simulink model "RoboticArm"  (R2023b)
settings: Solver=ode23t  StartTime=0.0  StopTime=100  RelTol=1e-3
model workspace: external: MATLAB File D:\Projects\RoboticArm\RoboticArm_DataFile1.m (data not in the file)
undefined symbols (not defined in the file or in its folder): dfdbk, dFilt, nfdbk, nFilt, smiData, ST, X, Y, Z
libraries: sm_lib x180, fl_lib x129, nesl_utility x69, ee_lib x39, slpidlib x25, simulink x18, SignalEditorBlockLib x1
(part 2 of 7)

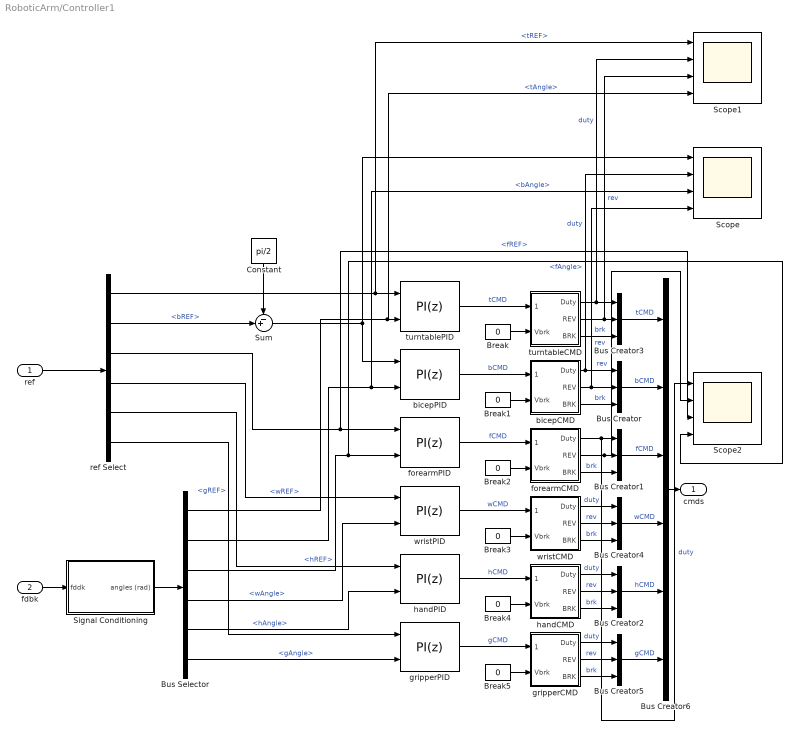
== system RoboticArm/Controller1 ==
  ref : Inport
  fdbk : Inport  Port=2
  Break{,1..5} (6 alike) : Constant  Value=0
  Bus Creator{,1..5} (6 alike) : BusCreator  Inputs=3
  Bus Creator6 : BusCreator  Inputs=6
  Bus Selector : BusSelector  OutputSignals=tAngle,bAngle,fAngle,wAngle,hAngle,gAngle
  Constant : Constant  Value=pi/2
  Scope : Scope  NumInputPorts=4
  Scope1 : Scope  NumInputPorts=4
  Scope2 : Scope  NumInputPorts=4
  Signal Conditioning : Subsystem
  Sum : Sum  Inputs=-+|
  bicepCMD : Subsystem
  bicepPID : slpidlib/PID Controller (2DOF)  Controller=PI  Form=Parallel  TimeDomain=Discrete-time  UseExternalTs=off  SampleTime=ST  IntegratorMethod=Forward Euler  FilterMethod=Backward Euler  ControllerParametersSource=internal  P=6  I=3  UseKiTs=off  D=2.0  N=25  UseFilter=on  b=1  c=1  TunerSelectOption=Transfer Function Based (PID Tuner App)  InitialConditionSource=internal  InitialConditionForIntegrator=0  InitialConditionForFilter=0  DifferentiatorICPrevScaledInput=0  ExternalReset=none  TrackingMode=off  Kt=1  LimitOutput=on  SatLimitsSource=internal  UpperSaturationLimit=5  LowerSaturationLimit=-5  LinearizeAsGain=on  AntiWindupMode=clamping  Kb=1  LimitIntegrator=off  UpperIntegratorSaturationLimit=inf  LowerIntegratorSaturationLimit=-inf  POutMin=[]  POutMax=[]  IOutMin=[]  IOutMax=[]  DOutMin=[]  DOutMax=[]  NOutMin=[]  NOutMax=[]  bOutMin=[]  bOutMax=[]  cOutMin=[]  cOutMax=[]  SumOutMin=[]  SumOutMax=[]  SaturationOutMin=[]  SaturationOutMax=[]  PParamMin=[]  PParamMax=[]  IParamMin=[]  IParamMax=[]  DParamMin=[]  DParamMax=[]  NParamMin=[]  NParamMax=[]  bParamMin=[]  bParamMax=[]  cParamMin=[]  cParamMax=[]  KbParamMin=[]  KbParamMax=[]  KtParamMin=[]  KtParamMax=[]  KbOutMin=[]  KbOutMax=[]  KtOutMin=[]  KtOutMax=[]  IntegratorOutMin=[]  IntegratorOutMax=[]  FilterOutMin=[]  FilterOutMax=[]  SumI1OutMin=[]  SumI1OutMax=[]  SumI2OutMin=[]  SumI2OutMax=[]  SumI3OutMin=[]  SumI3OutMax=[]  SumI4OutMin=[]  SumI4OutMax=[]  SumDOutMin=[]  SumDOutMax=[]  Sum1OutMin=[]  Sum1OutMax=[]  Sum2OutMin=[]  Sum2OutMax=[]  Sum3OutMin=[]  Sum3OutMax=[]  DifferentiatorOutMin=[]  DifferentiatorOutMax=[]  FilterDiffOutCoefMin=[]  FilterDiffOutCoefMax=[]  ReciprocalOutMin=[]  ReciprocalOutMax=[]  SumDenOutMin=[]  SumDenOutMax=[]  SumNumOutMin=[]  SumNumOutMax=[]  DivideOutMin=[]  DivideOutMax=[]  UdiffTsProdOutMin=[]  UdiffTsProdOutMax=[]  NTsProdOutMin=[]  NTsProdOutMax=[]  UintegralTsProdOutMin=[]  UintegralTsProdOutMax=[]  UngainTsProdOutMin=[]  UngainTsProdOutMax=[]  ClampingZeroOutDataTypeStr=Inherit: Inherit via back propagation  ClampingZeroOutMin=[]  ClampingZeroOutMax=[]  FilterDenConstantOutDataTypeStr=Inherit: Inherit via back propagation  FilterDenConstantOutMin=[]  FilterDenConstantOutMax=[]  PCopyOutDataTypeStr=Inherit: Inherit via back propagation  PCopyOutMin=[]  PCopyOutMax=[]  NCopyOutDataTypeStr=Inherit: Inherit via back propagation  NCopyOutMin=[]  NCopyOutMax=[]  IntegratorContinuousStateAttributes=''  IntegratorStateMustResolveToSignalObject=off  IntegratorRTWStateStorageClass=Auto  FilterContinuousStateAttributes=''  FilterStateMustResolveToSignalObject=off  FilterRTWStateStorageClass=Auto  ParallelPVariant=InternalParameters  IdealPVariant=Disabled  IVariant=InternalParameters  DVariant=Disabled  bVariant=InternalParameters  cVariant=Disabled  IntegratorVariant=Discrete  SatVariant=Enabled  AWVariant=DiscClampingParallel  PCopyVariant=Disabled  TRVariant=Disabled  FdbkBlocksVariant=Forward  IdealPFdbkVariant=Disabled  SatFdbkVariant=Disabled  DerivativeFilterVariant=Disabled  NVariant=Disabled  NCopyVariant=Disabled_SignalSpec  FilterICVariant=Disabled  IntegratorICVariant=InternalICs  ExternalResetVariant=Disabled  TRSumVariant=Passthrough  SumFdbkVariant=Disabled  SumVariant=Sum_PI  TsampFilterVariant=InternalTs  TsampNgainVariant=Passthrough  TsampIntegralVariant=Disabled_SignalSpec  ExternalSaturationOutDataTypeStr=Inherit: Same as second input
  forearmCMD : Subsystem
  forearmPID : slpidlib/PID Controller (2DOF)  Controller=PI  Form=Parallel  TimeDomain=Discrete-time  UseExternalTs=off  SampleTime=ST  IntegratorMethod=Forward Euler  FilterMethod=Backward Euler  ControllerParametersSource=internal  P=6  I=3  UseKiTs=off  D=2.0  N=25  UseFilter=on  b=1  c=1  TunerSelectOption=Transfer Function Based (PID Tuner App)  InitialConditionSource=internal  InitialConditionForIntegrator=0  InitialConditionForFilter=0  DifferentiatorICPrevScaledInput=0  ExternalReset=none  TrackingMode=off  Kt=1  LimitOutput=on  SatLimitsSource=internal  UpperSaturationLimit=5  LowerSaturationLimit=-5  LinearizeAsGain=on  AntiWindupMode=clamping  Kb=1  LimitIntegrator=off  UpperIntegratorSaturationLimit=inf  LowerIntegratorSaturationLimit=-inf  POutMin=[]  POutMax=[]  IOutMin=[]  IOutMax=[]  DOutMin=[]  DOutMax=[]  NOutMin=[]  NOutMax=[]  bOutMin=[]  bOutMax=[]  cOutMin=[]  cOutMax=[]  SumOutMin=[]  SumOutMax=[]  SaturationOutMin=[]  SaturationOutMax=[]  PParamMin=[]  PParamMax=[]  IParamMin=[]  IParamMax=[]  DParamMin=[]  DParamMax=[]  NParamMin=[]  NParamMax=[]  bParamMin=[]  bParamMax=[]  cParamMin=[]  cParamMax=[]  KbParamMin=[]  KbParamMax=[]  KtParamMin=[]  KtParamMax=[]  KbOutMin=[]  KbOutMax=[]  KtOutMin=[]  KtOutMax=[]  IntegratorOutMin=[]  IntegratorOutMax=[]  FilterOutMin=[]  FilterOutMax=[]  SumI1OutMin=[]  SumI1OutMax=[]  SumI2OutMin=[]  SumI2OutMax=[]  SumI3OutMin=[]  SumI3OutMax=[]  SumI4OutMin=[]  SumI4OutMax=[]  SumDOutMin=[]  SumDOutMax=[]  Sum1OutMin=[]  Sum1OutMax=[]  Sum2OutMin=[]  Sum2OutMax=[]  Sum3OutMin=[]  Sum3OutMax=[]  DifferentiatorOutMin=[]  DifferentiatorOutMax=[]  FilterDiffOutCoefMin=[]  FilterDiffOutCoefMax=[]  ReciprocalOutMin=[]  ReciprocalOutMax=[]  SumDenOutMin=[]  SumDenOutMax=[]  SumNumOutMin=[]  SumNumOutMax=[]  DivideOutMin=[]  DivideOutMax=[]  UdiffTsProdOutMin=[]  UdiffTsProdOutMax=[]  NTsProdOutMin=[]  NTsProdOutMax=[]  UintegralTsProdOutMin=[]  UintegralTsProdOutMax=[]  UngainTsProdOutMin=[]  UngainTsProdOutMax=[]  ClampingZeroOutDataTypeStr=Inherit: Inherit via back propagation  ClampingZeroOutMin=[]  ClampingZeroOutMax=[]  FilterDenConstantOutDataTypeStr=Inherit: Inherit via back propagation  FilterDenConstantOutMin=[]  FilterDenConstantOutMax=[]  PCopyOutDataTypeStr=Inherit: Inherit via back propagation  PCopyOutMin=[]  PCopyOutMax=[]  NCopyOutDataTypeStr=Inherit: Inherit via back propagation  NCopyOutMin=[]  NCopyOutMax=[]  IntegratorContinuousStateAttributes=''  IntegratorStateMustResolveToSignalObject=off  IntegratorRTWStateStorageClass=Auto  FilterContinuousStateAttributes=''  FilterStateMustResolveToSignalObject=off  FilterRTWStateStorageClass=Auto  ParallelPVariant=InternalParameters  IdealPVariant=Disabled  IVariant=InternalParameters  DVariant=Disabled  bVariant=InternalParameters  cVariant=Disabled  IntegratorVariant=Discrete  SatVariant=Enabled  AWVariant=DiscClampingParallel  PCopyVariant=Disabled  TRVariant=Disabled  FdbkBlocksVariant=Forward  IdealPFdbkVariant=Disabled  SatFdbkVariant=Disabled  DerivativeFilterVariant=Disabled  NVariant=Disabled  NCopyVariant=Disabled_SignalSpec  FilterICVariant=Disabled  IntegratorICVariant=InternalICs  ExternalResetVariant=Disabled  TRSumVariant=Passthrough  SumFdbkVariant=Disabled  SumVariant=Sum_PI  TsampFilterVariant=InternalTs  TsampNgainVariant=Passthrough  TsampIntegralVariant=Disabled_SignalSpec  ExternalSaturationOutDataTypeStr=Inherit: Same as second input
  gripperCMD : Subsystem
  gripperPID : slpidlib/PID Controller (2DOF)  Controller=PI  Form=Parallel  TimeDomain=Discrete-time  UseExternalTs=off  SampleTime=ST  IntegratorMethod=Forward Euler  FilterMethod=Backward Euler  ControllerParametersSource=internal  P=3  I=3  UseKiTs=off  D=2.0  N=25  UseFilter=on  b=1  c=1  TunerSelectOption=Transfer Function Based (PID Tuner App)  InitialConditionSource=internal  InitialConditionForIntegrator=0  InitialConditionForFilter=0  DifferentiatorICPrevScaledInput=0  ExternalReset=none  TrackingMode=off  Kt=1  LimitOutput=on  SatLimitsSource=internal  UpperSaturationLimit=5  LowerSaturationLimit=-5  LinearizeAsGain=on  AntiWindupMode=clamping  Kb=1  LimitIntegrator=off  UpperIntegratorSaturationLimit=inf  LowerIntegratorSaturationLimit=-inf  POutMin=[]  POutMax=[]  IOutMin=[]  IOutMax=[]  DOutMin=[]  DOutMax=[]  NOutMin=[]  NOutMax=[]  bOutMin=[]  bOutMax=[]  cOutMin=[]  cOutMax=[]  SumOutMin=[]  SumOutMax=[]  SaturationOutMin=[]  SaturationOutMax=[]  PParamMin=[]  PParamMax=[]  IParamMin=[]  IParamMax=[]  DParamMin=[]  DParamMax=[]  NParamMin=[]  NParamMax=[]  bParamMin=[]  bParamMax=[]  cParamMin=[]  cParamMax=[]  KbParamMin=[]  KbParamMax=[]  KtParamMin=[]  KtParamMax=[]  KbOutMin=[]  KbOutMax=[]  KtOutMin=[]  KtOutMax=[]  IntegratorOutMin=[]  IntegratorOutMax=[]  FilterOutMin=[]  FilterOutMax=[]  SumI1OutMin=[]  SumI1OutMax=[]  SumI2OutMin=[]  SumI2OutMax=[]  SumI3OutMin=[]  SumI3OutMax=[]  SumI4OutMin=[]  SumI4OutMax=[]  SumDOutMin=[]  SumDOutMax=[]  Sum1OutMin=[]  Sum1OutMax=[]  Sum2OutMin=[]  Sum2OutMax=[]  Sum3OutMin=[]  Sum3OutMax=[]  DifferentiatorOutMin=[]  DifferentiatorOutMax=[]  FilterDiffOutCoefMin=[]  FilterDiffOutCoefMax=[]  ReciprocalOutMin=[]  ReciprocalOutMax=[]  SumDenOutMin=[]  SumDenOutMax=[]  SumNumOutMin=[]  SumNumOutMax=[]  DivideOutMin=[]  DivideOutMax=[]  UdiffTsProdOutMin=[]  UdiffTsProdOutMax=[]  NTsProdOutMin=[]  NTsProdOutMax=[]  UintegralTsProdOutMin=[]  UintegralTsProdOutMax=[]  UngainTsProdOutMin=[]  UngainTsProdOutMax=[]  ClampingZeroOutDataTypeStr=Inherit: Inherit via back propagation  ClampingZeroOutMin=[]  ClampingZeroOutMax=[]  FilterDenConstantOutDataTypeStr=Inherit: Inherit via back propagation  FilterDenConstantOutMin=[]  FilterDenConstantOutMax=[]  PCopyOutDataTypeStr=Inherit: Inherit via back propagation  PCopyOutMin=[]  PCopyOutMax=[]  NCopyOutDataTypeStr=Inherit: Inherit via back propagation  NCopyOutMin=[]  NCopyOutMax=[]  IntegratorContinuousStateAttributes=''  IntegratorStateMustResolveToSignalObject=off  IntegratorRTWStateStorageClass=Auto  FilterContinuousStateAttributes=''  FilterStateMustResolveToSignalObject=off  FilterRTWStateStorageClass=Auto  ParallelPVariant=InternalParameters  IdealPVariant=Disabled  IVariant=InternalParameters  DVariant=Disabled  bVariant=InternalParameters  cVariant=Disabled  IntegratorVariant=Discrete  SatVariant=Enabled  AWVariant=DiscClampingParallel  PCopyVariant=Disabled  TRVariant=Disabled  FdbkBlocksVariant=Forward  IdealPFdbkVariant=Disabled  SatFdbkVariant=Disabled  DerivativeFilterVariant=Disabled  NVariant=Disabled  NCopyVariant=Disabled_SignalSpec  FilterICVariant=Disabled  IntegratorICVariant=InternalICs  ExternalResetVariant=Disabled  TRSumVariant=Passthrough  SumFdbkVariant=Disabled  SumVariant=Sum_PI  TsampFilterVariant=InternalTs  TsampNgainVariant=Passthrough  TsampIntegralVariant=Disabled_SignalSpec  ExternalSaturationOutDataTypeStr=Inherit: Same as second input
  handCMD : Subsystem
  handPID : slpidlib/PID Controller (2DOF)  Controller=PI  Form=Parallel  TimeDomain=Discrete-time  UseExternalTs=off  SampleTime=ST  IntegratorMethod=Forward Euler  FilterMethod=Backward Euler  ControllerParametersSource=internal  P=3  I=3  UseKiTs=off  D=2.0  N=25  UseFilter=on  b=1  c=1  TunerSelectOption=Transfer Function Based (PID Tuner App)  InitialConditionSource=internal  InitialConditionForIntegrator=0  InitialConditionForFilter=0  DifferentiatorICPrevScaledInput=0  ExternalReset=none  TrackingMode=off  Kt=1  LimitOutput=on  SatLimitsSource=internal  UpperSaturationLimit=5  LowerSaturationLimit=-5  LinearizeAsGain=on  AntiWindupMode=clamping  Kb=1  LimitIntegrator=off  UpperIntegratorSaturationLimit=inf  LowerIntegratorSaturationLimit=-inf  POutMin=[]  POutMax=[]  IOutMin=[]  IOutMax=[]  DOutMin=[]  DOutMax=[]  NOutMin=[]  NOutMax=[]  bOutMin=[]  bOutMax=[]  cOutMin=[]  cOutMax=[]  SumOutMin=[]  SumOutMax=[]  SaturationOutMin=[]  SaturationOutMax=[]  PParamMin=[]  PParamMax=[]  IParamMin=[]  IParamMax=[]  DParamMin=[]  DParamMax=[]  NParamMin=[]  NParamMax=[]  bParamMin=[]  bParamMax=[]  cParamMin=[]  cParamMax=[]  KbParamMin=[]  KbParamMax=[]  KtParamMin=[]  KtParamMax=[]  KbOutMin=[]  KbOutMax=[]  KtOutMin=[]  KtOutMax=[]  IntegratorOutMin=[]  IntegratorOutMax=[]  FilterOutMin=[]  FilterOutMax=[]  SumI1OutMin=[]  SumI1OutMax=[]  SumI2OutMin=[]  SumI2OutMax=[]  SumI3OutMin=[]  SumI3OutMax=[]  SumI4OutMin=[]  SumI4OutMax=[]  SumDOutMin=[]  SumDOutMax=[]  Sum1OutMin=[]  Sum1OutMax=[]  Sum2OutMin=[]  Sum2OutMax=[]  Sum3OutMin=[]  Sum3OutMax=[]  DifferentiatorOutMin=[]  DifferentiatorOutMax=[]  FilterDiffOutCoefMin=[]  FilterDiffOutCoefMax=[]  ReciprocalOutMin=[]  ReciprocalOutMax=[]  SumDenOutMin=[]  SumDenOutMax=[]  SumNumOutMin=[]  SumNumOutMax=[]  DivideOutMin=[]  DivideOutMax=[]  UdiffTsProdOutMin=[]  UdiffTsProdOutMax=[]  NTsProdOutMin=[]  NTsProdOutMax=[]  UintegralTsProdOutMin=[]  UintegralTsProdOutMax=[]  UngainTsProdOutMin=[]  UngainTsProdOutMax=[]  ClampingZeroOutDataTypeStr=Inherit: Inherit via back propagation  ClampingZeroOutMin=[]  ClampingZeroOutMax=[]  FilterDenConstantOutDataTypeStr=Inherit: Inherit via back propagation  FilterDenConstantOutMin=[]  FilterDenConstantOutMax=[]  PCopyOutDataTypeStr=Inherit: Inherit via back propagation  PCopyOutMin=[]  PCopyOutMax=[]  NCopyOutDataTypeStr=Inherit: Inherit via back propagation  NCopyOutMin=[]  NCopyOutMax=[]  IntegratorContinuousStateAttributes=''  IntegratorStateMustResolveToSignalObject=off  IntegratorRTWStateStorageClass=Auto  FilterContinuousStateAttributes=''  FilterStateMustResolveToSignalObject=off  FilterRTWStateStorageClass=Auto  ParallelPVariant=InternalParameters  IdealPVariant=Disabled  IVariant=InternalParameters  DVariant=Disabled  bVariant=InternalParameters  cVariant=Disabled  IntegratorVariant=Discrete  SatVariant=Enabled  AWVariant=DiscClampingParallel  PCopyVariant=Disabled  TRVariant=Disabled  FdbkBlocksVariant=Forward  IdealPFdbkVariant=Disabled  SatFdbkVariant=Disabled  DerivativeFilterVariant=Disabled  NVariant=Disabled  NCopyVariant=Disabled_SignalSpec  FilterICVariant=Disabled  IntegratorICVariant=InternalICs  ExternalResetVariant=Disabled  TRSumVariant=Passthrough  SumFdbkVariant=Disabled  SumVariant=Sum_PI  TsampFilterVariant=InternalTs  TsampNgainVariant=Passthrough  TsampIntegralVariant=Disabled_SignalSpec  ExternalSaturationOutDataTypeStr=Inherit: Same as second input
  ref Select : BusSelector  OutputSignals=tREF,bREF,fREF,wREF,hREF,gREF
  turntableCMD : Subsystem
  turntablePID : slpidlib/PID Controller (2DOF)  Controller=PI  Form=Parallel  TimeDomain=Discrete-time  UseExternalTs=off  SampleTime=ST  IntegratorMethod=Forward Euler  FilterMethod=Backward Euler  ControllerParametersSource=internal  P=3  I=3  UseKiTs=off  D=2.0  N=25  UseFilter=on  b=1  c=1  TunerSelectOption=Transfer Function Based (PID Tuner App)  InitialConditionSource=internal  InitialConditionForIntegrator=0  InitialConditionForFilter=0  DifferentiatorICPrevScaledInput=0  ExternalReset=none  TrackingMode=off  Kt=1  LimitOutput=on  SatLimitsSource=internal  UpperSaturationLimit=5  LowerSaturationLimit=-5  LinearizeAsGain=on  AntiWindupMode=clamping  Kb=1  LimitIntegrator=off  UpperIntegratorSaturationLimit=inf  LowerIntegratorSaturationLimit=-inf  POutMin=[]  POutMax=[]  IOutMin=[]  IOutMax=[]  DOutMin=[]  DOutMax=[]  NOutMin=[]  NOutMax=[]  bOutMin=[]  bOutMax=[]  cOutMin=[]  cOutMax=[]  SumOutMin=[]  SumOutMax=[]  SaturationOutMin=[]  SaturationOutMax=[]  PParamMin=[]  PParamMax=[]  IParamMin=[]  IParamMax=[]  DParamMin=[]  DParamMax=[]  NParamMin=[]  NParamMax=[]  bParamMin=[]  bParamMax=[]  cParamMin=[]  cParamMax=[]  KbParamMin=[]  KbParamMax=[]  KtParamMin=[]  KtParamMax=[]  KbOutMin=[]  KbOutMax=[]  KtOutMin=[]  KtOutMax=[]  IntegratorOutMin=[]  IntegratorOutMax=[]  FilterOutMin=[]  FilterOutMax=[]  SumI1OutMin=[]  SumI1OutMax=[]  SumI2OutMin=[]  SumI2OutMax=[]  SumI3OutMin=[]  SumI3OutMax=[]  SumI4OutMin=[]  SumI4OutMax=[]  SumDOutMin=[]  SumDOutMax=[]  Sum1OutMin=[]  Sum1OutMax=[]  Sum2OutMin=[]  Sum2OutMax=[]  Sum3OutMin=[]  Sum3OutMax=[]  DifferentiatorOutMin=[]  DifferentiatorOutMax=[]  FilterDiffOutCoefMin=[]  FilterDiffOutCoefMax=[]  ReciprocalOutMin=[]  ReciprocalOutMax=[]  SumDenOutMin=[]  SumDenOutMax=[]  SumNumOutMin=[]  SumNumOutMax=[]  DivideOutMin=[]  DivideOutMax=[]  UdiffTsProdOutMin=[]  UdiffTsProdOutMax=[]  NTsProdOutMin=[]  NTsProdOutMax=[]  UintegralTsProdOutMin=[]  UintegralTsProdOutMax=[]  UngainTsProdOutMin=[]  UngainTsProdOutMax=[]  ClampingZeroOutDataTypeStr=Inherit: Inherit via back propagation  ClampingZeroOutMin=[]  ClampingZeroOutMax=[]  FilterDenConstantOutDataTypeStr=Inherit: Inherit via back propagation  FilterDenConstantOutMin=[]  FilterDenConstantOutMax=[]  PCopyOutDataTypeStr=Inherit: Inherit via back propagation  PCopyOutMin=[]  PCopyOutMax=[]  NCopyOutDataTypeStr=Inherit: Inherit via back propagation  NCopyOutMin=[]  NCopyOutMax=[]  IntegratorContinuousStateAttributes=''  IntegratorStateMustResolveToSignalObject=off  IntegratorRTWStateStorageClass=Auto  FilterContinuousStateAttributes=''  FilterStateMustResolveToSignalObject=off  FilterRTWStateStorageClass=Auto  ParallelPVariant=InternalParameters  IdealPVariant=Disabled  IVariant=InternalParameters  DVariant=Disabled  bVariant=InternalParameters  cVariant=Disabled  IntegratorVariant=Discrete  SatVariant=Enabled  AWVariant=DiscClampingParallel  PCopyVariant=Disabled  TRVariant=Disabled  FdbkBlocksVariant=Forward  IdealPFdbkVariant=Disabled  SatFdbkVariant=Disabled  DerivativeFilterVariant=Disabled  NVariant=Disabled  NCopyVariant=Disabled_SignalSpec  FilterICVariant=Disabled  IntegratorICVariant=InternalICs  ExternalResetVariant=Disabled  TRSumVariant=Passthrough  SumFdbkVariant=Disabled  SumVariant=Sum_PI  TsampFilterVariant=InternalTs  TsampNgainVariant=Passthrough  TsampIntegralVariant=Disabled_SignalSpec  ExternalSaturationOutDataTypeStr=Inherit: Same as second input
  wristCMD : Subsystem
  wristPID : slpidlib/PID Controller (2DOF)  Controller=PI  Form=Parallel  TimeDomain=Discrete-time  UseExternalTs=off  SampleTime=ST  IntegratorMethod=Forward Euler  FilterMethod=Backward Euler  ControllerParametersSource=internal  P=3  I=3  UseKiTs=off  D=2.0  N=25  UseFilter=on  b=1  c=1  TunerSelectOption=Transfer Function Based (PID Tuner App)  InitialConditionSource=internal  InitialConditionForIntegrator=0  InitialConditionForFilter=0  DifferentiatorICPrevScaledInput=0  ExternalReset=none  TrackingMode=off  Kt=1  LimitOutput=on  SatLimitsSource=internal  UpperSaturationLimit=5  LowerSaturationLimit=-5  LinearizeAsGain=on  AntiWindupMode=clamping  Kb=1  LimitIntegrator=off  UpperIntegratorSaturationLimit=inf  LowerIntegratorSaturationLimit=-inf  POutMin=[]  POutMax=[]  IOutMin=[]  IOutMax=[]  DOutMin=[]  DOutMax=[]  NOutMin=[]  NOutMax=[]  bOutMin=[]  bOutMax=[]  cOutMin=[]  cOutMax=[]  SumOutMin=[]  SumOutMax=[]  SaturationOutMin=[]  SaturationOutMax=[]  PParamMin=[]  PParamMax=[]  IParamMin=[]  IParamMax=[]  DParamMin=[]  DParamMax=[]  NParamMin=[]  NParamMax=[]  bParamMin=[]  bParamMax=[]  cParamMin=[]  cParamMax=[]  KbParamMin=[]  KbParamMax=[]  KtParamMin=[]  KtParamMax=[]  KbOutMin=[]  KbOutMax=[]  KtOutMin=[]  KtOutMax=[]  IntegratorOutMin=[]  IntegratorOutMax=[]  FilterOutMin=[]  FilterOutMax=[]  SumI1OutMin=[]  SumI1OutMax=[]  SumI2OutMin=[]  SumI2OutMax=[]  SumI3OutMin=[]  SumI3OutMax=[]  SumI4OutMin=[]  SumI4OutMax=[]  SumDOutMin=[]  SumDOutMax=[]  Sum1OutMin=[]  Sum1OutMax=[]  Sum2OutMin=[]  Sum2OutMax=[]  Sum3OutMin=[]  Sum3OutMax=[]  DifferentiatorOutMin=[]  DifferentiatorOutMax=[]  FilterDiffOutCoefMin=[]  FilterDiffOutCoefMax=[]  ReciprocalOutMin=[]  ReciprocalOutMax=[]  SumDenOutMin=[]  SumDenOutMax=[]  SumNumOutMin=[]  SumNumOutMax=[]  DivideOutMin=[]  DivideOutMax=[]  UdiffTsProdOutMin=[]  UdiffTsProdOutMax=[]  NTsProdOutMin=[]  NTsProdOutMax=[]  UintegralTsProdOutMin=[]  UintegralTsProdOutMax=[]  UngainTsProdOutMin=[]  UngainTsProdOutMax=[]  ClampingZeroOutDataTypeStr=Inherit: Inherit via back propagation  ClampingZeroOutMin=[]  ClampingZeroOutMax=[]  FilterDenConstantOutDataTypeStr=Inherit: Inherit via back propagation  FilterDenConstantOutMin=[]  FilterDenConstantOutMax=[]  PCopyOutDataTypeStr=Inherit: Inherit via back propagation  PCopyOutMin=[]  PCopyOutMax=[]  NCopyOutDataTypeStr=Inherit: Inherit via back propagation  NCopyOutMin=[]  NCopyOutMax=[]  IntegratorContinuousStateAttributes=''  IntegratorStateMustResolveToSignalObject=off  IntegratorRTWStateStorageClass=Auto  FilterContinuousStateAttributes=''  FilterStateMustResolveToSignalObject=off  FilterRTWStateStorageClass=Auto  ParallelPVariant=InternalParameters  IdealPVariant=Disabled  IVariant=InternalParameters  DVariant=Disabled  bVariant=InternalParameters  cVariant=Disabled  IntegratorVariant=Discrete  SatVariant=Enabled  AWVariant=DiscClampingParallel  PCopyVariant=Disabled  TRVariant=Disabled  FdbkBlocksVariant=Forward  IdealPFdbkVariant=Disabled  SatFdbkVariant=Disabled  DerivativeFilterVariant=Disabled  NVariant=Disabled  NCopyVariant=Disabled_SignalSpec  FilterICVariant=Disabled  IntegratorICVariant=InternalICs  ExternalResetVariant=Disabled  TRSumVariant=Passthrough  SumFdbkVariant=Disabled  SumVariant=Sum_PI  TsampFilterVariant=InternalTs  TsampNgainVariant=Passthrough  TsampIntegralVariant=Disabled_SignalSpec  ExternalSaturationOutDataTypeStr=Inherit: Same as second input
  cmds : Outport  VectorParamsAs1DForOutWhenUnconnected=off
  wires:
  Constant/1 -> Sum/1
  Sum/1 -> Scope/1, bicepPID/1
  ref Select/2 -> Sum/2  "<bREF>"
  Bus Selector/2 -> Scope/3, bicepPID/2  "<bAngle>"
  Signal Conditioning/1(angles (rad)) -> Bus Selector/1
  fdbk/1 -> Signal Conditioning/1(fddk)
  ref Select/6 -> gripperPID/1  "<gREF>"
  ref Select/5 -> handPID/1  "<hREF>"
  ref Select/4 -> wristPID/1  "<wREF>"
  ref Select/3 -> forearmPID/1, Scope2/3  "<fREF>"
  ref Select/1 -> turntablePID/1, Scope1/1  "<tREF>"
  Bus Selector/1 -> turntablePID/2, Scope1/4  "<tAngle>"
  Bus Selector/3 -> forearmPID/2, Scope2/4  "<fAngle>"
  Bus Selector/4 -> wristPID/2  "<wAngle>"
  Bus Selector/5 -> handPID/2  "<hAngle>"
  Bus Selector/6 -> gripperPID/2  "<gAngle>"
  Bus Creator6/1 -> cmds/1
  Bus Creator/1 -> Bus Creator6/2  "bCMD"
  Bus Creator5/1 -> Bus Creator6/6  "gCMD"
  Break5/1 -> gripperCMD/2(Vbrk)
  gripperPID/1 -> gripperCMD/1(Vcmd)  "gCMD"
  gripperCMD/1(Duty) -> Bus Creator5/1  "duty"
  gripperCMD/3(BRK) -> Bus Creator5/3  "brk"
  gripperCMD/2(REV) -> Bus Creator5/2  "rev"
  Bus Creator4/1 -> Bus Creator6/4  "wCMD"
  Break3/1 -> wristCMD/2(Vbrk)
  wristPID/1 -> wristCMD/1(Vcmd)  "wCMD"
  wristCMD/1(Duty) -> Bus Creator4/1  "duty"
  wristCMD/3(BRK) -> Bus Creator4/3  "brk"
  wristCMD/2(REV) -> Bus Creator4/2  "rev"
  Bus Creator3/1 -> Bus Creator6/1  "tCMD"
  Break/1 -> turntableCMD/2(Vbrk)
  turntablePID/1 -> turntableCMD/1(Vcmd)  "tCMD"
  turntableCMD/3(BRK) -> Bus Creator3/3  "brk"
  turntableCMD/2(REV) -> Bus Creator3/2, Scope1/3  "rev"
  turntableCMD/1(Duty) -> Bus Creator3/1, Scope1/2  "duty"
  ref/1 -> ref Select/1
  Bus Creator2/1 -> Bus Creator6/5  "hCMD"
  Bus Creator1/1 -> Bus Creator6/3  "fCMD"
  Break4/1 -> handCMD/2(Vbrk)
  handPID/1 -> handCMD/1(Vcmd)  "hCMD"
  Break2/1 -> forearmCMD/2(Vbrk)
  forearmPID/1 -> forearmCMD/1(Vcmd)  "fCMD"
  Break1/1 -> bicepCMD/2(Vbrk)
  bicepPID/1 -> bicepCMD/1(Vcmd)  "bCMD"
  handCMD/1(Duty) -> Bus Creator2/1  "duty"
  handCMD/3(BRK) -> Bus Creator2/3  "brk"
  handCMD/2(REV) -> Bus Creator2/2  "rev"
  forearmCMD/3(BRK) -> Bus Creator1/3  "brk"
  forearmCMD/2(REV) -> Bus Creator1/2, Scope2/2  "rev"
  forearmCMD/1(Duty) -> Bus Creator1/1, Scope2/1  "duty"
  bicepCMD/3(BRK) -> Bus Creator/3  "brk"
  bicepCMD/2(REV) -> Bus Creator/2, Scope/4  "rev"
  bicepCMD/1(Duty) -> Scope/2, Bus Creator/1  "duty"

== system RoboticArm/Desired Angles ==
  Bicep : Constant  Value=-1.656111915345903
  Bus Creator : BusCreator  Inputs=7
  Forearn : Constant  Value=2.617730895324456
  Gain{,1..5} (6 alike) : Gain  Gain=pi/180
  Gripper : Constant  Value=100
  Gripper Base : Constant  Value=-0.2492901370839746
  Hand : Constant  Value=-52.96002450101879
  Turntable : Constant  Value=-1.656111915345903
  Wrist : Constant  Value=-0.2492901370839746
  . : Outport
  wires:
  Gripper Base/1 -> Gain5/1
  Hand/1 -> Gain4/1
  Wrist/1 -> Gain3/1
  Forearn/1 -> Gain2/1
  Bicep/1 -> Gain1/1
  Turntable/1 -> Gain/1
  Bus Creator/1 -> ./1  "REF"
  Gain/1 -> Bus Creator/1  "tREF"
  Gain4/1 -> Bus Creator/5  "hREF"
  Gain5/1 -> Bus Creator/6  "gREF"
  Gain2/1 -> Bus Creator/3  "fREF"
  Gain3/1 -> Bus Creator/4  "wREF"
  Gain1/1 -> Bus Creator/2  "bREF"
  Gripper/1 -> Bus Creator/7  "gsREF"

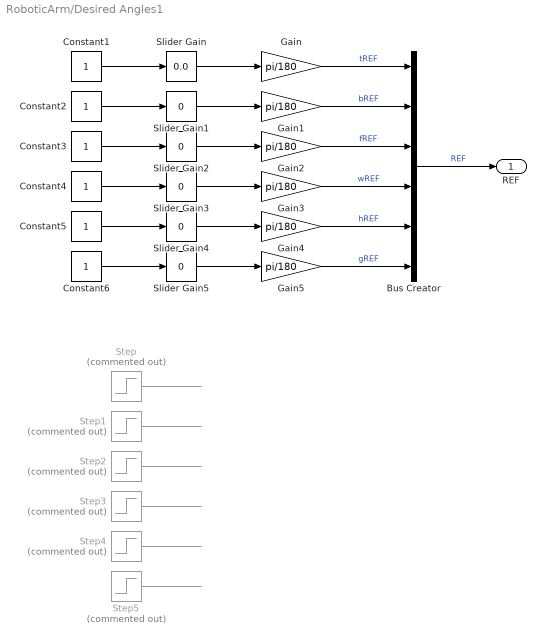
== system RoboticArm/Desired Angles1 ==
  Bus Creator : BusCreator  Inputs=6
  Constant{1..6} (6 alike) : Constant
  Gain{,1..5} (6 alike) : Gain  Gain=pi/180
  Slider Gain : simulink/Math Operations/Slider Gain  gain=0.0  low=-180  high=180
  Slider Gain{1..5} (5 alike) : simulink/Math Operations/Slider Gain  gain=0  low=-180  high=180
  Step{,2..5} (5 alike) : Step  Commented=on  After=80  SampleTime=ST
  Step1 : Step  Commented=on  Before=90  After=80  SampleTime=ST
  REF : Outport
  wires:
  Slider Gain5/1 -> Gain5/1
  Constant6/1 -> Slider Gain5/1
  Constant5/1 -> Slider Gain4/1
  Slider Gain4/1 -> Gain4/1
  Slider Gain3/1 -> Gain3/1
  Constant4/1 -> Slider Gain3/1
  Constant3/1 -> Slider Gain2/1
  Slider Gain2/1 -> Gain2/1
  Slider Gain1/1 -> Gain1/1
  Constant2/1 -> Slider Gain1/1
  Constant1/1 -> Slider Gain/1
  Slider Gain/1 -> Gain/1
  Step1/1 -> ?
  Step3/1 -> ?
  Step4/1 -> ?
  Step2/1 -> ?
  Step5/1 -> ?
  Step/1 -> ?
  Bus Creator/1 -> REF/1  "REF"
  Gain/1 -> Bus Creator/1  "tREF"
  Gain4/1 -> Bus Creator/5  "hREF"
  Gain5/1 -> Bus Creator/6  "gREF"
  Gain2/1 -> Bus Creator/3  "fREF"
  Gain3/1 -> Bus Creator/4  "wREF"
  Gain1/1 -> Bus Creator/2  "bREF"

== system RoboticArm/Desired Anglesa ==
  Bus Creator : BusCreator  Inputs=6
  Constant{1..6} (6 alike) : Constant
  Gain{,1..5} (6 alike) : Gain  Gain=pi/180
  Slider Gain : simulink/Math Operations/Slider Gain  gain=0.0  low=-180  high=180
  Slider Gain{1..5} (5 alike) : simulink/Math Operations/Slider Gain  gain=0  low=-180  high=180
  REF : Outport
  wires:
  Slider Gain5/1 -> Gain5/1
  Constant6/1 -> Slider Gain5/1
  Constant5/1 -> Slider Gain4/1
  Slider Gain4/1 -> Gain4/1
  Slider Gain3/1 -> Gain3/1
  Constant4/1 -> Slider Gain3/1
  Constant3/1 -> Slider Gain2/1
  Slider Gain2/1 -> Gain2/1
  Slider Gain1/1 -> Gain1/1
  Constant2/1 -> Slider Gain1/1
  Constant1/1 -> Slider Gain/1
  Slider Gain/1 -> Gain/1
  Bus Creator/1 -> REF/1  "REF"
  Gain/1 -> Bus Creator/1  "tREF"
  Gain4/1 -> Bus Creator/5  "hREF"
  Gain5/1 -> Bus Creator/6  "gREF"
  Gain2/1 -> Bus Creator/3  "fREF"
  Gain3/1 -> Bus Creator/4  "wREF"
  Gain1/1 -> Bus Creator/2  "bREF"

== system RoboticArm/Plant ==
  CMDs : Inport
  Bus Creator : BusCreator  Inputs=6
  Bus Selector : BusSelector  OutputSignals=tCMD,bCMD,fCMD,wCMD,hCMD,gCMD
  DC motors : Subsystem
  Mechanical Design : Subsystem
  PS-Simulink Converter{,1..5} (6 alike) : nesl_utility/PS-Simulink Converter  PhysicalDomain=network_engine_domain  SubClassName=ps_output  LeftPortType=input  RightPortType=output  PseudoPeriodic=off  Frequencies=[]  VectorFormat=inherit  Unit=inherit  AffineConversion=off
  Angles : Outport
  wires:
  PS-Simulink Converter4/1 -> Bus Creator/5  "hAngle"
  Bus Selector/6 -> DC motors/6(gCMD)  "<gCMD>"
  PS-Simulink Converter1/1 -> Bus Creator/2  "bAngle"
  Bus Selector/4 -> DC motors/4(wCMD)  "<wCMD>"
  Bus Selector/5 -> DC motors/5(hCMD)  "<hCMD>"
  Bus Selector/1 -> DC motors/1(tCMD)  "<tCMD>"
  PS-Simulink Converter5/1 -> Bus Creator/6  "gAngle"
  PS-Simulink Converter2/1 -> Bus Creator/3  "fAngle"
  PS-Simulink Converter3/1 -> Bus Creator/4  "wAngle"
  PS-Simulink Converter/1 -> Bus Creator/1  "tAngle"
  Bus Selector/2 -> DC motors/2(bCMD)  "<bCMD>"
  Bus Selector/3 -> DC motors/3(fCMD)  "<fCMD>"
  CMDs/1 -> Bus Selector/1
  Bus Creator/1 -> Angles/1
  connections:
  Mechanical Design/LConn1 -- DC motors/RConn1
  Mechanical Design/LConn2 -- DC motors/RConn2
  Mechanical Design/LConn3 -- DC motors/RConn3
  Mechanical Design/LConn5 -- DC motors/RConn5
  Mechanical Design/LConn6 -- DC motors/RConn6
  Mechanical Design/LConn7 -- DC motors/RConn7
  Mechanical Design/LConn8 -- DC motors/RConn8
  Mechanical Design/LConn9 -- DC motors/RConn9
  Mechanical Design/LConn10 -- DC motors/RConn10
  Mechanical Design/LConn11 -- DC motors/RConn11
  Mechanical Design/LConn12 -- DC motors/RConn12
  Mechanical Design/RConn1 -- PS-Simulink Converter/LConn1
  Mechanical Design/RConn2 -- PS-Simulink Converter1/LConn1
  Mechanical Design/RConn3 -- PS-Simulink Converter2/LConn1
  Mechanical Design/RConn4 -- PS-Simulink Converter3/LConn1
  Mechanical Design/RConn5 -- PS-Simulink Converter4/LConn1
  Mechanical Design/RConn6 -- PS-Simulink Converter5/LConn1
  Mechanical Design/LConn4 -- DC motors/RConn4

== system RoboticArm/Plant1 ==
  CMDs : Inport
  Bus Creator : BusCreator  Inputs=6
  Bus Selector : BusSelector  OutputSignals=tREF,bREF,fREF,wREF,hREF,gREF
  PS-Simulink Converter{,1..5} (6 alike) : nesl_utility/PS-Simulink Converter  PhysicalDomain=network_engine_domain  SubClassName=ps_output  LeftPortType=input  RightPortType=output  PseudoPeriodic=off  Frequencies=[]  VectorFormat=inherit  Unit=inherit  AffineConversion=off
  Simulink-PS Converter{,1..5} (6 alike) : nesl_utility/Simulink-PS Converter  PhysicalDomain=network_engine_domain  SubClassName=ps_input  LeftPortType=input  RightPortType=output  PseudoPeriodic=off  Frequencies=[]  NoiseDistribution=none  NoiseParameters=[]  Unit=1  AffineConversion=off  FilteringAndDerivatives=provide  SimscapeFilterOrder=1  InputFilterTimeConstant=0.001  UdotUserProvided=0
  Subsystem1 : Subsystem
  Angles : Outport
  wires:
  Bus Creator/1 -> Angles/1
  CMDs/1 -> Bus Selector/1
  PS-Simulink Converter/1 -> Bus Creator/1  "tAngle"
  PS-Simulink Converter3/1 -> Bus Creator/4  "wAngle"
  PS-Simulink Converter2/1 -> Bus Creator/3  "fAngle"
  PS-Simulink Converter5/1 -> Bus Creator/6  "gAngle"
  PS-Simulink Converter1/1 -> Bus Creator/2  "bAngle"
  PS-Simulink Converter4/1 -> Bus Creator/5  "hAngle"
  Bus Selector/6 -> Simulink-PS Converter/1  "<gREF>"
  Bus Selector/5 -> Simulink-PS Converter1/1  "<hREF>"
  Bus Selector/4 -> Simulink-PS Converter2/1  "<wREF>"
  Bus Selector/1 -> Simulink-PS Converter5/1  "<tREF>"
  Bus Selector/2 -> Simulink-PS Converter4/1  "<bREF>"
  Bus Selector/3 -> Simulink-PS Converter3/1  "<fREF>"
  connections:
  PS-Simulink Converter/LConn1 -- Subsystem1/RConn1
  Subsystem1/RConn4 -- PS-Simulink Converter3/LConn1
  Subsystem1/RConn6 -- PS-Simulink Converter5/LConn1
  Subsystem1/RConn3 -- PS-Simulink Converter2/LConn1
  PS-Simulink Converter1/LConn1 -- Subsystem1/RConn2
  PS-Simulink Converter4/LConn1 -- Subsystem1/RConn5
  Simulink-PS Converter/RConn1 -- Subsystem1/LConn6
  Simulink-PS Converter1/RConn1 -- Subsystem1/LConn5
  Simulink-PS Converter2/RConn1 -- Subsystem1/LConn4
  Simulink-PS Converter5/RConn1 -- Subsystem1/LConn1
  Simulink-PS Converter4/RConn1 -- Subsystem1/LConn2
  Simulink-PS Converter3/RConn1 -- Subsystem1/LConn3

== system RoboticArm/Reference Angle Test Vectors ==
  Bus Creator : BusCreator  Inputs=6
  Gain{,1..5} (6 alike) : Gain  Gain=pi/180
  Joint Angle Test Vectors : SignalEditorBlockLib/Signal Editor  FileName=dcst_robotarm_JointAngleSignalEditorData.mat  ActiveScenario=Two_Points_Test_1  ActiveSignal=Gripper Angle (deg)  IsBus=off  OutputBusObjectStr=Bus: BusObject  SampleTime=0  OutputAfterFinalValue=Extrapolation  Unit=inherit  PreserveSignalName=on  ApplySigPropsToAllScenarios=on  ApplySigPropsToAllSignals=off
  ref : Outport  VectorParamsAs1DForOutWhenUnconnected=off
  wires:
  Joint Angle Test Vectors/1 -> Gain/1
  Joint Angle Test Vectors/2 -> Gain1/1
  Joint Angle Test Vectors/3 -> Gain2/1
  Joint Angle Test Vectors/4 -> Gain3/1
  Joint Angle Test Vectors/5 -> Gain4/1
  Joint Angle Test Vectors/6 -> Gain5/1
  Bus Creator/1 -> ref/1
  Gain/1 -> Bus Creator/1  "tREF"
  Gain1/1 -> Bus Creator/2  "bREF"
  Gain2/1 -> Bus Creator/3  "fREF"
  Gain3/1 -> Bus Creator/4  "wREF"
  Gain4/1 -> Bus Creator/5  "hREF"
  Gain5/1 -> Bus Creator/6  "gREF"

== system RoboticArm/Simulation Angles ==
  Bus Creator : BusCreator  Inputs=6
  Constant{1..6} (6 alike) : Constant
  Gain{,1..5} (6 alike) : Gain  Gain=pi/180
  Slider Gain : simulink/Math Operations/Slider Gain  gain=-90.0  low=-180  high=180
  Slider Gain{1..5} (5 alike) : simulink/Math Operations/Slider Gain  gain=0  low=-180  high=180
  REF : Outport
  wires:
  Gain1/1 -> Bus Creator/2  "bREF"
  Gain3/1 -> Bus Creator/4  "wREF"
  Gain2/1 -> Bus Creator/3  "fREF"
  Gain5/1 -> Bus Creator/6  "gREF"
  Gain4/1 -> Bus Creator/5  "hREF"
  Gain/1 -> Bus Creator/1  "tREF"
  Bus Creator/1 -> REF/1  "REF"
  Slider Gain/1 -> Gain/1
  Constant1/1 -> Slider Gain/1
  Constant2/1 -> Slider Gain1/1
  Slider Gain1/1 -> Gain1/1
  Slider Gain2/1 -> Gain2/1
  Constant3/1 -> Slider Gain2/1
  Constant4/1 -> Slider Gain3/1
  Slider Gain3/1 -> Gain3/1
  Slider Gain4/1 -> Gain4/1
  Constant5/1 -> Slider Gain4/1
  Constant6/1 -> Slider Gain5/1
  Slider Gain5/1 -> Gain5/1

== system RoboticArm/Subsystem ==
  cmds : Inport
  Bus Creator : BusCreator  Inputs=6
  Bus Selector : BusSelector  OutputSignals=tCMD,bCMD,fCMD,wCMD,hCMD,gCMD,gsREF
  DC Motors : Subsystem
      mask Display: image('MultiServos.jpg',[0.25 0.1 0.5 0.8])
  Mechanical design : Subsystem
      settings: PortSchema="{\"entries\":[{\"content\":{\"sides\":[{\"content\":{\"connectorIds\":[\"LConn1\",\"LConn2\",\"LConn3\",\"LConn4\",\"LConn5\",\"LConn6\",\"LConn7\",\"LConn8\",\"LConn9\",\"LConn10\",\"LConn11\",\"LConn12\",\"In1\"]},\"type\":\"ConnectorPlacement.EquallySpacedRectSide\",\"uuid\":\"f71d7aae-a57b-4430-aa21-449d4269cfdf\"},{\"content\":{\"connectorIds\":[\"RConn1\",\"RConn2\",\"RConn3\",\"RConn4\",\"RConn5\",\"RConn6\"],\"side\":\"RIGHT\"},\"type\":\"ConnectorPlacement.EquallySpacedRectSide\",\"uuid\":\"bfce3b01-c64c-4762-9bf8-a0f7b486b75d\"},{\"content\":{\"side\":\"TOP\"},\"type\":\"ConnectorPlacement.EquallySpacedRectSide\",\"uuid\":\"bdc0640b-aaa1-4bb7-b324-502ee0804488\"}]},\"type\":\"ConnectorPlacement.EquallySpacedConnector\",\"uuid\":\"700e3925-c040-4176-a732-a9f385af8522\"}],\"packageUris\":[\"http://schema.mathworks.com/mf0/Connector/R2020b\"],\"version\":\"1.0\"}"
      mask Display: image('Screenshot 2024-04-15 211552.png');
  PS-Simulink Converter{,1..5} (6 alike) : nesl_utility/PS-Simulink Converter  PhysicalDomain=network_engine_domain  SubClassName=ps_output  LeftPortType=input  RightPortType=output  PseudoPeriodic=off  Frequencies=[]  VectorFormat=1-D array  Unit=rad  AffineConversion=off
  angles : Outport  VectorParamsAs1DForOutWhenUnconnected=off
  wires:
  Bus Selector/3 -> DC Motors/3(fCMD)  "<fCMD>"
  PS-Simulink Converter5/1 -> Bus Creator/6  "gAngle"
  Bus Selector/5 -> DC Motors/5(hCMD)  "<hCMD>"
  Bus Selector/7 -> Mechanical design/1(In1)  "<gsREF>"
  Bus Selector/1 -> DC Motors/1(tCMD)  "<tCMD>"
  Bus Selector/6 -> DC Motors/6(gCMD)  "<gCMD>"
  Bus Selector/4 -> DC Motors/4(wCMD)  "<wCMD>"
  cmds/1 -> Bus Selector/1
  Bus Creator/1 -> angles/1
  Bus Selector/2 -> DC Motors/2(bCMD)  "<bCMD>"
  PS-Simulink Converter1/1 -> Bus Creator/2  "bAngle"
  PS-Simulink Converter2/1 -> Bus Creator/3  "fAngle"
  PS-Simulink Converter3/1 -> Bus Creator/4  "wAngle"
  PS-Simulink Converter4/1 -> Bus Creator/5  "hAngle"
  PS-Simulink Converter/1 -> Bus Creator/1  "tAngle"
  connections:
  Mechanical design/LConn8 -- DC Motors/RConn8
  Mechanical design/LConn1 -- DC Motors/RConn1
  PS-Simulink Converter1/LConn1 -- Mechanical design/RConn2
  Mechanical design/LConn6 -- DC Motors/RConn6
  Mechanical design/LConn3 -- DC Motors/RConn3
  Mechanical design/LConn12 -- DC Motors/RConn12
  Mechanical design/LConn9 -- DC Motors/RConn9
  Mechanical design/RConn6 -- PS-Simulink Converter5/LConn1
  PS-Simulink Converter4/LConn1 -- Mechanical design/RConn5
  Mechanical design/LConn5 -- DC Motors/RConn5
  Mechanical design/LConn2 -- DC Motors/RConn2
  Mechanical design/LConn4 -- DC Motors/RConn4
  Mechanical design/LConn7 -- DC Motors/RConn7
  PS-Simulink Converter3/LConn1 -- Mechanical design/RConn4
  Mechanical design/LConn10 -- DC Motors/RConn10
  Mechanical design/LConn11 -- DC Motors/RConn11
  Mechanical design/RConn3 -- PS-Simulink Converter2/LConn1
  PS-Simulink Converter/LConn1 -- Mechanical design/RConn1

== system RoboticArm/Subsystem1 ==
  REF : Inport
  Feedback : Inport  Port=2
  Bus Creator7 : BusCreator  Inputs=6
  Bus Selector : BusSelector  OutputSignals=tREF,bREF,fREF,wREF,hREF,gREF
  Bus Selector1 : BusSelector  OutputSignals=tAngle,bAngle,fAngle,wAngle,hAngle,gAngle
  PID Controller (2DOF)2 : slpidlib/PID Controller (2DOF)  Commented=on  Controller=PID  Form=Parallel  TimeDomain=Discrete-time  UseExternalTs=off  SampleTime=ST  IntegratorMethod=Forward Euler  FilterMethod=Forward Euler  ControllerParametersSource=internal  P=1.1776  I=1.3387  UseKiTs=off  D=0.001  N=100  UseFilter=on  b=1  c=1  TunerSelectOption=Frequency Response Based  InitialConditionSource=internal  InitialConditionForIntegrator=0  InitialConditionForFilter=0  DifferentiatorICPrevScaledInput=0  ExternalReset=none  TrackingMode=off  Kt=1  LimitOutput=off  SatLimitsSource=internal  UpperSaturationLimit=inf  LowerSaturationLimit=-inf  LinearizeAsGain=on  AntiWindupMode=none  Kb=1  LimitIntegrator=off  UpperIntegratorSaturationLimit=inf  LowerIntegratorSaturationLimit=-inf  POutMin=[]  POutMax=[]  IOutMin=[]  IOutMax=[]  DOutMin=[]  DOutMax=[]  NOutMin=[]  NOutMax=[]  bOutMin=[]  bOutMax=[]  cOutMin=[]  cOutMax=[]  SumOutMin=[]  SumOutMax=[]  SaturationOutMin=[]  SaturationOutMax=[]  PParamMin=[]  PParamMax=[]  IParamMin=[]  IParamMax=[]  DParamMin=[]  DParamMax=[]  NParamMin=[]  NParamMax=[]  bParamMin=[]  bParamMax=[]  cParamMin=[]  cParamMax=[]  KbParamMin=[]  KbParamMax=[]  KtParamMin=[]  KtParamMax=[]  KbOutMin=[]  KbOutMax=[]  KtOutMin=[]  KtOutMax=[]  IntegratorOutMin=[]  IntegratorOutMax=[]  FilterOutMin=[]  FilterOutMax=[]  SumI1OutMin=[]  SumI1OutMax=[]  SumI2OutMin=[]  SumI2OutMax=[]  SumI3OutMin=[]  SumI3OutMax=[]  SumI4OutMin=[]  SumI4OutMax=[]  SumDOutMin=[]  SumDOutMax=[]  Sum1OutMin=[]  Sum1OutMax=[]  Sum2OutMin=[]  Sum2OutMax=[]  Sum3OutMin=[]  Sum3OutMax=[]  DifferentiatorOutMin=[]  DifferentiatorOutMax=[]  FilterDiffOutCoefMin=[]  FilterDiffOutCoefMax=[]  ReciprocalOutMin=[]  ReciprocalOutMax=[]  SumDenOutMin=[]  SumDenOutMax=[]  SumNumOutMin=[]  SumNumOutMax=[]  DivideOutMin=[]  DivideOutMax=[]  UdiffTsProdOutMin=[]  UdiffTsProdOutMax=[]  NTsProdOutMin=[]  NTsProdOutMax=[]  UintegralTsProdOutMin=[]  UintegralTsProdOutMax=[]  UngainTsProdOutMin=[]  UngainTsProdOutMax=[]  ClampingZeroOutDataTypeStr=Inherit: Inherit via back propagation  ClampingZeroOutMin=[]  ClampingZeroOutMax=[]  FilterDenConstantOutDataTypeStr=Inherit: Inherit via back propagation  FilterDenConstantOutMin=[]  FilterDenConstantOutMax=[]  PCopyOutDataTypeStr=Inherit: Inherit via back propagation  PCopyOutMin=[]  PCopyOutMax=[]  NCopyOutDataTypeStr=Inherit: Inherit via back propagation  NCopyOutMin=[]  NCopyOutMax=[]  IntegratorContinuousStateAttributes=''  IntegratorStateMustResolveToSignalObject=off  IntegratorRTWStateStorageClass=Auto  FilterContinuousStateAttributes=''  FilterStateMustResolveToSignalObject=off  FilterRTWStateStorageClass=Auto  ParallelPVariant=InternalParameters  IdealPVariant=Disabled  IVariant=InternalParameters  DVariant=InternalParameters  bVariant=InternalParameters  cVariant=InternalParameters  IntegratorVariant=Discrete  SatVariant=Disabled  AWVariant=Passthrough  PCopyVariant=Disabled  TRVariant=Disabled  FdbkBlocksVariant=Forward  IdealPFdbkVariant=Disabled  SatFdbkVariant=Disabled  DerivativeFilterVariant=ForwardEulerFilter  NVariant=InternalParameters  NCopyVariant=Disabled  FilterICVariant=InternalICsFilter  IntegratorICVariant=InternalICs  ExternalResetVariant=Disabled  TRSumVariant=Passthrough  SumFdbkVariant=Disabled  SumVariant=Sum_PID  TsampFilterVariant=InternalTs  TsampNgainVariant=Passthrough  TsampIntegralVariant=Disabled_SignalSpec  ExternalSaturationOutDataTypeStr=Inherit: Same as second input
  Transfer Function : Subsystem  Commented=on
  CMDs : Outport
  wires:
  Feedback/1 -> Bus Selector1/1
  Bus Creator7/1 -> CMDs/1
  REF/1 -> Bus Selector/1
  Bus Selector/1 -> Bus Creator7/1  "<tREF>"
  Bus Selector/2 -> Bus Creator7/2  "<bREF>"
  Bus Selector/3 -> Bus Creator7/3  "<fREF>"
  Bus Selector/4 -> Bus Creator7/4  "<wREF>"
  Bus Selector/5 -> Bus Creator7/5  "<hREF>"
  Bus Selector/6 -> Bus Creator7/6  "<gREF>"

== system RoboticArm/Subsystem2 ==
  Bus Creator : BusCreator  Inputs=6
  Gain{,1..5} (6 alike) : Gain  Gain=pi/180
  Step{,2..5} (5 alike) : Step  After=80  SampleTime=ST
  Step1 : Step  Before=90  After=80  SampleTime=ST
  REF : Outport
  wires:
  Step5/1 -> Gain5/1
  Step4/1 -> Gain4/1
  Step3/1 -> Gain3/1
  Step2/1 -> Gain2/1
  Step1/1 -> Gain1/1
  Step/1 -> Gain/1
  Bus Creator/1 -> REF/1  "REF"
  Gain/1 -> Bus Creator/1  "tREF"
  Gain4/1 -> Bus Creator/5  "hREF"
  Gain5/1 -> Bus Creator/6  "gREF"
  Gain2/1 -> Bus Creator/3  "fREF"
  Gain3/1 -> Bus Creator/4  "wREF"
  Gain1/1 -> Bus Creator/2  "bREF"

== system RoboticArm/Control Panel /Bicep  ==

== system RoboticArm/Control Panel /Forearm ==

== system RoboticArm/Control Panel /Gripper ==

== system RoboticArm/Control Panel /Gripper base ==

== system RoboticArm/Control Panel /Hand ==

== system RoboticArm/Control Panel /Turntable ==

== system RoboticArm/Control Panel /Wrist ==

== system RoboticArm/Control System/Subsystem1 ==
  signal : Inport
  Abs : Abs  SaturateOnIntegerOverflow=off
  Fcn : Fcn  Expr=u(1)<0
  Gain : Gain  Gain=5
  "[0...5]" : Saturate  UpperLimit=5  LowerLimit=0
  duty : Outport
  rev : Outport  Port=2
  wires:
  signal/1 -> Fcn/1, Abs/1
  Abs/1 -> "[0...5]"/1
  Fcn/1 -> Gain/1
  Gain/1 -> rev/1
  "[0...5]"/1 -> duty/1

== system RoboticArm/Control System/Subsystem2 ==
  signal : Inport
  Abs : Abs  SaturateOnIntegerOverflow=off
  Fcn : Fcn  Expr=u(1)<0
  Gain : Gain  Gain=5
  "[0...5]" : Saturate  UpperLimit=5  LowerLimit=0
  duty : Outport
  rev : Outport  Port=2
  wires:
  "[0...5]"/1 -> duty/1
  Gain/1 -> rev/1
  Fcn/1 -> Gain/1
  Abs/1 -> "[0...5]"/1
  signal/1 -> Abs/1, Fcn/1

== system RoboticArm/Control System/Subsystem3 ==
  signal : Inport
  Abs : Abs  SaturateOnIntegerOverflow=off
  Fcn : Fcn  Expr=u(1)<0
  Gain : Gain  Gain=5
  "[0...5]" : Saturate  UpperLimit=5  LowerLimit=0
  duty : Outport
  rev : Outport  Port=2
  wires:
  signal/1 -> Fcn/1, Abs/1
  Abs/1 -> "[0...5]"/1
  Fcn/1 -> Gain/1
  Gain/1 -> rev/1
  "[0...5]"/1 -> duty/1

== system RoboticArm/Control System/Subsystem4 ==
  signal : Inport
  Abs : Abs  SaturateOnIntegerOverflow=off
  Fcn : Fcn  Expr=u(1)<0
  Gain : Gain  Gain=5
  "[0...5]" : Saturate  UpperLimit=5  LowerLimit=0
  duty : Outport
  rev : Outport  Port=2
  wires:
  "[0...5]"/1 -> duty/1
  Gain/1 -> rev/1
  Fcn/1 -> Gain/1
  Abs/1 -> "[0...5]"/1
  signal/1 -> Abs/1, Fcn/1

== system RoboticArm/Control System/Subsystem5 ==
  signal : Inport
  Abs : Abs  SaturateOnIntegerOverflow=off
  Fcn : Fcn  Expr=u(1)<0
  Gain : Gain  Gain=5
  "[0...5]" : Saturate  UpperLimit=5  LowerLimit=0
  duty : Outport
  rev : Outport  Port=2
  wires:
  signal/1 -> Fcn/1, Abs/1
  Abs/1 -> "[0...5]"/1
  Fcn/1 -> Gain/1
  Gain/1 -> rev/1
  "[0...5]"/1 -> duty/1

== system RoboticArm/Control System/Subsystem6 ==
  signal : Inport
  Abs : Abs  SaturateOnIntegerOverflow=off
  Fcn : Fcn  Expr=u(1)<0
  Gain : Gain  Gain=5
  "[0...5]" : Saturate  UpperLimit=5  LowerLimit=0
  duty : Outport
  rev : Outport  Port=2
  wires:
  "[0...5]"/1 -> duty/1
  Gain/1 -> rev/1
  Fcn/1 -> Gain/1
  Abs/1 -> "[0...5]"/1
  signal/1 -> Abs/1, Fcn/1

== system RoboticArm/Control System/Transfer Function ==
  Fdbk : Inport
  Bus Creator6 : BusCreator  Inputs=6
  Bus Selector2 : BusSelector  OutputSignals=tAngle,bAngle,fAngle,wAngle,hAngle,gAngle
  Constant1 : Constant  Value=pi/2
  Discrete Transfer Fcn{,1..5} (6 alike) : DiscreteTransferFcn  Numerator=nFilt  Denominator=dFilt  SampleTime=ST
  Sum1 : Sum  Inputs=|+-
  Angles : Outport
  wires:
  Sum1/1 -> Discrete Transfer Fcn1/1
  Discrete Transfer Fcn2/1 -> Bus Creator6/3  "fAngle"
  Discrete Transfer Fcn/1 -> Bus Creator6/1  "tAngle"
  Discrete Transfer Fcn3/1 -> Bus Creator6/4  "wAngle"
  Discrete Transfer Fcn4/1 -> Bus Creator6/5  "hAngle"
  Fdbk/1 -> Bus Selector2/1
  Discrete Transfer Fcn5/1 -> Bus Creator6/6  "gAngle"
  Discrete Transfer Fcn1/1 -> Bus Creator6/2  "bAngle"
  Constant1/1 -> Sum1/2
  Bus Selector2/2 -> Sum1/1  "<bAngle>"
  Bus Selector2/4 -> Discrete Transfer Fcn3/1  "<wAngle>"
  Bus Selector2/1 -> Discrete Transfer Fcn/1  "<tAngle>"
  Bus Creator6/1 -> Angles/1
  Bus Selector2/3 -> Discrete Transfer Fcn2/1  "<fAngle>"
  Bus Selector2/6 -> Discrete Transfer Fcn5/1  "<gAngle>"
  Bus Selector2/5 -> Discrete Transfer Fcn4/1  "<hAngle>"

== system RoboticArm/Control System/brk value ==
  Constant1 : Constant  Value=0
  brk : Outport
  wires:
  Constant1/1 -> brk/1  "brk"

== system RoboticArm/Control System1/Subsystem1 ==
  signal : Inport
  Abs : Abs  SaturateOnIntegerOverflow=off
  Fcn : Fcn  Expr=u(1)<0
  Gain : Gain  Gain=5
  "[0...5]" : Saturate  UpperLimit=5  LowerLimit=0
  duty : Outport
  rev : Outport  Port=2
  wires:
  "[0...5]"/1 -> duty/1
  Gain/1 -> rev/1
  Fcn/1 -> Gain/1
  Abs/1 -> "[0...5]"/1
  signal/1 -> Abs/1, Fcn/1

== system RoboticArm/Control System1/Subsystem2 ==
  signal : Inport
  Abs : Abs  SaturateOnIntegerOverflow=off
  Fcn : Fcn  Expr=u(1)<0
  Gain : Gain  Gain=5
  "[0...5]" : Saturate  UpperLimit=5  LowerLimit=0
  duty : Outport
  rev : Outport  Port=2
  wires:
  signal/1 -> Fcn/1, Abs/1
  Abs/1 -> "[0...5]"/1
  Fcn/1 -> Gain/1
  Gain/1 -> rev/1
  "[0...5]"/1 -> duty/1

== system RoboticArm/Control System1/Subsystem3 ==
  signal : Inport
  Abs : Abs  SaturateOnIntegerOverflow=off
  Fcn : Fcn  Expr=u(1)<0
  Gain : Gain  Gain=5
  "[0...5]" : Saturate  UpperLimit=5  LowerLimit=0
  duty : Outport
  rev : Outport  Port=2
  wires:
  "[0...5]"/1 -> duty/1
  Gain/1 -> rev/1
  Fcn/1 -> Gain/1
  Abs/1 -> "[0...5]"/1
  signal/1 -> Abs/1, Fcn/1

== system RoboticArm/Control System1/Subsystem4 ==
  signal : Inport
  Abs : Abs  SaturateOnIntegerOverflow=off
  Fcn : Fcn  Expr=u(1)<0
  Gain : Gain  Gain=5
  "[0...5]" : Saturate  UpperLimit=5  LowerLimit=0
  duty : Outport
  rev : Outport  Port=2
  wires:
  signal/1 -> Fcn/1, Abs/1
  Abs/1 -> "[0...5]"/1
  Fcn/1 -> Gain/1
  Gain/1 -> rev/1
  "[0...5]"/1 -> duty/1

== system RoboticArm/Control System1/Subsystem5 ==
  signal : Inport
  Abs : Abs  SaturateOnIntegerOverflow=off
  Fcn : Fcn  Expr=u(1)<0
  Gain : Gain  Gain=5
  "[0...5]" : Saturate  UpperLimit=5  LowerLimit=0
  duty : Outport
  rev : Outport  Port=2
  wires:
  "[0...5]"/1 -> duty/1
  Gain/1 -> rev/1
  Fcn/1 -> Gain/1
  Abs/1 -> "[0...5]"/1
  signal/1 -> Abs/1, Fcn/1

== system RoboticArm/Control System1/Subsystem6 ==
  signal : Inport
  Abs : Abs  SaturateOnIntegerOverflow=off
  Fcn : Fcn  Expr=u(1)<0
  Gain : Gain  Gain=5
  "[0...5]" : Saturate  UpperLimit=5  LowerLimit=0
  duty : Outport
  rev : Outport  Port=2
  wires:
  signal/1 -> Fcn/1, Abs/1
  Abs/1 -> "[0...5]"/1
  Fcn/1 -> Gain/1
  Gain/1 -> rev/1
  "[0...5]"/1 -> duty/1

== system RoboticArm/Control System1/Transfer Function ==
  Fdbk : Inport
  Bus Creator6 : BusCreator  Inputs=6
  Bus Selector2 : BusSelector  OutputSignals=tAngle,bAngle,fAngle,wAngle,hAngle,gAngle
  Constant1 : Constant  Value=pi/2
  Discrete Transfer Fcn{,1..5} (6 alike) : DiscreteTransferFcn  Numerator=nFilt  Denominator=dFilt  SampleTime=ST
  Sum1 : Sum  Inputs=|+-
  Angles : Outport
  wires:
  Bus Selector2/5 -> Discrete Transfer Fcn4/1  "<hAngle>"
  Bus Selector2/6 -> Discrete Transfer Fcn5/1  "<gAngle>"
  Bus Selector2/3 -> Discrete Transfer Fcn2/1  "<fAngle>"
  Bus Creator6/1 -> Angles/1
  Bus Selector2/1 -> Discrete Transfer Fcn/1  "<tAngle>"
  Bus Selector2/4 -> Discrete Transfer Fcn3/1  "<wAngle>"
  Bus Selector2/2 -> Sum1/1  "<bAngle>"
  Constant1/1 -> Sum1/2
  Discrete Transfer Fcn1/1 -> Bus Creator6/2  "bAngle"
  Discrete Transfer Fcn5/1 -> Bus Creator6/6  "gAngle"
  Fdbk/1 -> Bus Selector2/1
  Discrete Transfer Fcn4/1 -> Bus Creator6/5  "hAngle"
  Discrete Transfer Fcn3/1 -> Bus Creator6/4  "wAngle"
  Discrete Transfer Fcn/1 -> Bus Creator6/1  "tAngle"
  Discrete Transfer Fcn2/1 -> Bus Creator6/3  "fAngle"
  Sum1/1 -> Discrete Transfer Fcn1/1

== system RoboticArm/Control System3/Subsystem1 ==
  signal : Inport
  Abs : Abs  SaturateOnIntegerOverflow=off
  Fcn : Fcn  Expr=u(1)<0
  Gain : Gain  Gain=5
  "[0...5]" : Saturate  UpperLimit=5  LowerLimit=0
  duty : Outport
  rev : Outport  Port=2
  wires:
  signal/1 -> Fcn/1, Abs/1
  Abs/1 -> "[0...5]"/1
  Fcn/1 -> Gain/1
  Gain/1 -> rev/1
  "[0...5]"/1 -> duty/1

== system RoboticArm/Control System3/Subsystem2 ==
  signal : Inport
  Abs : Abs  SaturateOnIntegerOverflow=off
  Fcn : Fcn  Expr=u(1)<0
  Gain : Gain  Gain=5
  "[0...5]" : Saturate  UpperLimit=5  LowerLimit=0
  duty : Outport
  rev : Outport  Port=2
  wires:
  "[0...5]"/1 -> duty/1
  Gain/1 -> rev/1
  Fcn/1 -> Gain/1
  Abs/1 -> "[0...5]"/1
  signal/1 -> Abs/1, Fcn/1
